simulink model "traffic_light"  (R2024b)
settings: Solver=ode45  StartTime=0.0  StopTime=10.0  RelTol=1e-3
settings Model: Creator=HP  LastModifiedBy=HP

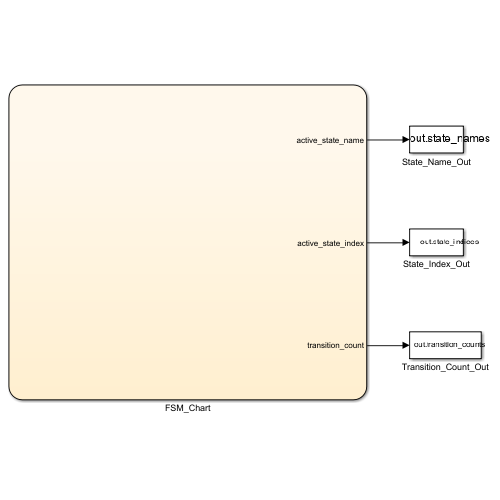
[thumbnail: Simulink's stored preview of the top-level diagram]
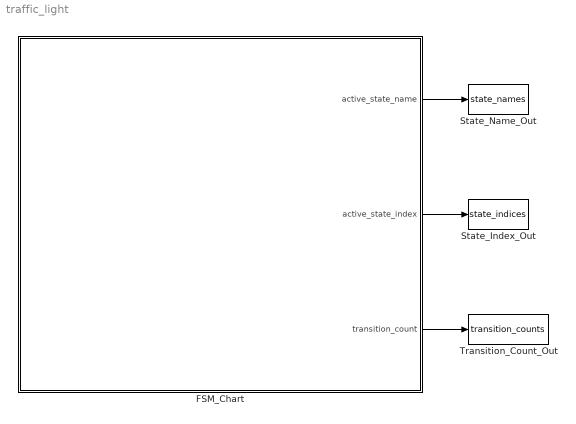
== system traffic_light ==
  FSM_Chart : Stateflow chart  TreatAsAtomicUnit=on
  State_Index_Out : ToWorkspace  VariableName=state_indices  SaveFormat=Timeseries  SampleTime=-1
  State_Name_Out : ToWorkspace  VariableName=state_names  SaveFormat=Timeseries  SampleTime=-1
  Transition_Count_Out : ToWorkspace  VariableName=transition_counts  SaveFormat=Timeseries  SampleTime=-1
  wires:
  FSM_Chart/1(active_state_name) -> State_Name_Out/1
  FSM_Chart/2(active_state_index) -> State_Index_Out/1
  FSM_Chart/3(transition_count) -> Transition_Count_Out/1

== stateflow chart traffic_light/FSM_Chart ==
  state entry_1 active_state_name = 'Yellow'; active_state_index = 2;\nentry: try; print(''Light is YELLOW''); timer_start_tick = current_tick; event_sent = False; catch; end;\nduring: try; YELLOW_DURATION = 2; if not event_sent and current_tick >= timer_start_tick + YELLOW_DURATION:;   sm.send(''timer_yellow_expired'');   event_sent = True; catch; end;
    settings: description=Traffic light is yellow. Prepare to stop or proceed with caution.
  state entry_2 active_state_name = 'Red'; active_state_index = 3;\nentry: try; print(''Light is RED''); timer_start_tick = current_tick; event_sent = False; catch; end;\nduring: try; RED_DURATION = 5; if not event_sent and current_tick >= timer_start_tick + RED_DURATION:;   sm.send(''timer_red_expired'');   event_sent = True; catch; end;
    settings: description=Traffic light is red. Stop.
  state entry_ active_state_name = 'Green'; active_state_index = 1;\nentry: try; print(''Light is GREEN''); timer_start_tick = current_tick; event_sent = False; catch; end;\nduring: try; GREEN_DURATION = 5; if not event_sent and current_tick >= timer_start_tick + GREEN_DURATION:;   sm.send(''timer_green_expired'');   event_sent = True; catch; end;
    settings: description=Traffic light is green. Go.
  (default) -> entry_2 active_state_name = 'Red'; active_state_index = 3;\nentry: try; print(''Light is RED''); timer_start_tick = current_tick; event_sent = False; catch; end;\nduring: try; RED_DURATION = 5; if not event_sent and current_tick >= timer_start_tick + RED_DURATION:;   sm.send(''timer_red_expired'');   event_sent = True; catch; end; : [trans_count_local = 0]
    settings: description=Initial transition to Red
  entry_1 active_state_name = 'Yellow'; active_state_index = 2;\nentry: try; print(''Light is YELLOW''); timer_start_tick = current_tick; event_sent = False; catch; end;\nduring: try; YELLOW_DURATION = 2; if not event_sent and current_tick >= timer_start_tick + YELLOW_DURATION:;   sm.send(''timer_yellow_expired'');   event_sent = True; catch; end; -> entry_2 active_state_name = 'Red'; active_state_index = 3;\nentry: try; print(''Light is RED''); timer_start_tick = current_tick; event_sent = False; catch; end;\nduring: try; RED_DURATION = 5; if not event_sent and current_tick >= timer_start_tick + RED_DURATION:;   sm.send(''timer_red_expired'');   event_sent = True; catch; end; : timer_yellow_expired /{try; print(''Transition: Yellow to Red''); catch; end; trans_count_local = trans_count_local + 1; transition_count = trans_count_local}
    settings: description=Transition from Yellow to Red
  entry_ active_state_name = 'Green'; active_state_index = 1;\nentry: try; print(''Light is GREEN''); timer_start_tick = current_tick; event_sent = False; catch; end;\nduring: try; GREEN_DURATION = 5; if not event_sent and current_tick >= timer_start_tick + GREEN_DURATION:;   sm.send(''timer_green_expired'');   event_sent = True; catch; end; -> entry_1 active_state_name = 'Yellow'; active_state_index = 2;\nentry: try; print(''Light is YELLOW''); timer_start_tick = current_tick; event_sent = False; catch; end;\nduring: try; YELLOW_DURATION = 2; if not event_sent and current_tick >= timer_start_tick + YELLOW_DURATION:;   sm.send(''timer_yellow_expired'');   event_sent = True; catch; end; : timer_green_expired /{try; print(''Transition: Green to Yellow''); catch; end; trans_count_local = trans_count_local + 1; transition_count = trans_count_local}
    settings: description=Transition from Green to Yellow
  entry_2 active_state_name = 'Red'; active_state_index = 3;\nentry: try; print(''Light is RED''); timer_start_tick = current_tick; event_sent = False; catch; end;\nduring: try; RED_DURATION = 5; if not event_sent and current_tick >= timer_start_tick + RED_DURATION:;   sm.send(''timer_red_expired'');   event_sent = True; catch; end; -> entry_ active_state_name = 'Green'; active_state_index = 1;\nentry: try; print(''Light is GREEN''); timer_start_tick = current_tick; event_sent = False; catch; end;\nduring: try; GREEN_DURATION = 5; if not event_sent and current_tick >= timer_start_tick + GREEN_DURATION:;   sm.send(''timer_green_expired'');   event_sent = True; catch; end; : timer_red_expired /{try; print(''Transition: Red to Green''); catch; end; trans_count_local = trans_count_local + 1; transition_count = trans_count_local}
    settings: description=Transition from Red to Green
  data: active_state_name output string; active_state_index output uint8; transition_count output uint32; trans_count_local local uint32
